simulink model "dezim_2"  (Simulink 7.8)
settings: Solver=FixedStepDiscrete  SolverMode=MultiTasking  StartTime=0.0  StopTime=1  RelTol=1e-3
undefined symbols (not defined in the file or in its folder): get
libraries: dspsigops x2, dspsnks4 x2, dsparch4 x1
settings Model: Creator=svenhoffmann  LastModifiedBy=josef  ExtModeAutoUpdateStatusClock=off
settings DataIOCC: SignalLoggingName=sigsOut
settings DebuggingCC: SaveWithParameterizedLinksMsg=none  SignalResolutionControl=TryResolveAllWithWarning  SolverPrmCheckMsg=none  MultiTaskDSMMsg=warning  MultiTaskCondExecSysMsg=none  StrictBusMsg=None
settings HardwareCC: TargetUnknown=on
settings RTWCC: IncludeERTFirstTime=on

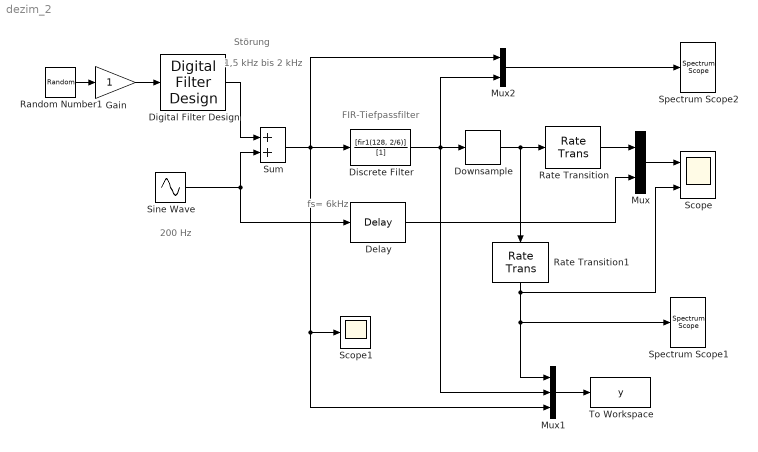
== system dezim_2 ==
  note: Störung
  note: 200 Hz
  note: 1,5 kHz bis
      | 2 kHz
  note: fs=
      | 6kHz
  note: FIR-Tiefpassfilter
  Delay : dspsigops/Delay  InputProcessing=Inherited (this choice will be removed - see release notes)  dly_unit=Samples  delay=64  ic_detail=off  dif_ic_for_ch=off  dif_ic_for_dly=off  ic=0  reset_popup=None
  Digital Filter Design : dsparch4/Digital Filter Design  mwdsp_browser_bugfix_var=off
  Discrete Filter : DiscreteFilter  Numerator=[fir1(128, 2/6)]  Denominator=[1]  SampleTime=1/6000
  Downsample : dspsigops/Downsample  N=3  phase=0  InputProcessing=Inherited (this choice will be removed - see release notes)  RateOptions=Enforce single-rate processing  smode=Allow multirate  fmode=Maintain input frame size  ic=0
  Gain : Gain  SaturateOnIntegerOverflow=on  OutDataTypeStr=Inherit: Same as input  ParamDataTypeStr=Inherit: Same as input
  Mux : Mux  Inputs=2
  Mux1 : Mux  Inputs=3
  Mux2 : Mux  Inputs=2
  Random Number1 : RandomNumber  Seed=1739  SampleTime=1/6000
  Rate Transition : RateTransition
  Rate Transition1 : RateTransition
  Scope : Scope  NumInputPorts=2
      settings: YMin=-1.2~-5  YMax=1.1~5
  Scope1 : Scope
  Sine Wave : Sin  Frequency=2*pi*200  SampleTime=1/6000
  Spectrum Scope1 : dspsnks4/Spectrum Scope  ScopeProperties=off  Domain=Frequency  HorizSpan=1  UseBuffer=on  BufferSize=256  Overlap=64  TreatMby1Signals=M channels  inpFftLenInherit=off  FFTlength=128  numAvg=10  DisplayProperties=off  AxisGrid=on  Memory=off  FrameNumber=on  AxisLegend=off  AxisZoom=off  OpenScopeAtSimStart=on  OpenScopeImmediately=off  FigPos=get(0,'defaultfigureposition')  AxisProperties=on  XUnits=Hertz  XRange=[0...Fs]  XDisplay=0  InheritXIncr=off  XIncr=1/6000  XLabel=Samples  XLimit=Auto  YUnits=dBW/Hertz  XMax=1  XMin=0  YLabel=Magnitude, dB  LineProperties=off  wintypeSpecScope=Hann  RsSpecScope=50  betaSpecScope=5  winsampSpecScope=Periodic  XAxisParamsVer=6.8  isFrameUpgraded=on
      settings: YMin=-125.6782  YMax=-22.0978
  Spectrum Scope2 : dspsnks4/Spectrum Scope  ScopeProperties=off  Domain=Frequency  HorizSpan=1  UseBuffer=on  BufferSize=256  Overlap=64  TreatMby1Signals=M channels  inpFftLenInherit=off  FFTlength=128  numAvg=10  DisplayProperties=off  AxisGrid=on  Memory=off  FrameNumber=on  AxisLegend=off  AxisZoom=off  OpenScopeAtSimStart=on  OpenScopeImmediately=off  FigPos=get(0,'defaultfigureposition')  AxisProperties=on  XUnits=Hertz  XRange=[0...Fs]  XDisplay=0  InheritXIncr=off  XIncr=1/6000  XLabel=Samples  XLimit=Auto  YUnits=dBW/Hertz  XMax=1  XMin=0  YLabel=Magnitude, dB  LineProperties=off  wintypeSpecScope=Hann  RsSpecScope=50  betaSpecScope=5  winsampSpecScope=Periodic  XAxisParamsVer=6.8  isFrameUpgraded=on
      settings: YMin=-168.3645  YMax=-21.964
  Sum : Sum  SaturateOnIntegerOverflow=on
  To Workspace : ToWorkspace  VariableName=y  SampleTime=-1  SaveFormat=Array
  wires:
  Random Number1/1 -> Gain/1
  Sine Wave/1 -> Sum/2, Delay/1
  Gain/1 -> Digital Filter Design/1
  Digital Filter Design/1 -> Sum/1
  Sum/1 -> Discrete Filter/1, Mux2/1, Mux1/3, Scope1/1
  Discrete Filter/1 -> Downsample/1, Mux2/2, Mux1/2
  Downsample/1 -> Rate Transition/1, Rate Transition1/1
  Mux/1 -> Scope/1
  Delay/1 -> Mux/2
  Mux1/1 -> To Workspace/1
  Mux2/1 -> Spectrum Scope2/1
  Rate Transition/1 -> Mux/1
  Rate Transition1/1 -> Mux1/1, Spectrum Scope1/1, Scope/2
